simulink model "PID_Closed_Loop_2"  (R2023b)
settings: Solver=VariableStepAuto  StartTime=0.0  StopTime=100  FixedStep=0.1  RelTol=1e-05
values from neighbouring files (symbols this model uses):
  F_max = 1.0    (= 1)    [Parameters.m]    (also in Parameters_.m)
  J = 1    [Parameters.m]    (also in Parameters_.m = 0.0178)
  Kd = 5    [Parameters.m]    (also in Parameters_.m = 8)
  KI = 5    [Parameters.m]    (also in Parameters_.m = 2)
  Kp = 8    [Parameters.m]    (also in Parameters_.m)
  L = 0.160    (= 0.16)    [Parameters.m]    (also in Parameters_.m = 0.41)
  m = 2    [Parameters.m]    (also in Parameters_.m = 2.05)
  r = 0.033    [Parameters.m]    (also in Parameters_.m = 0.1)
libraries: slpidlib x2
settings Model: Creator=yosse  LastModifiedBy=DELL
settings DebuggingCC: AlgebraicLoopMsg=none

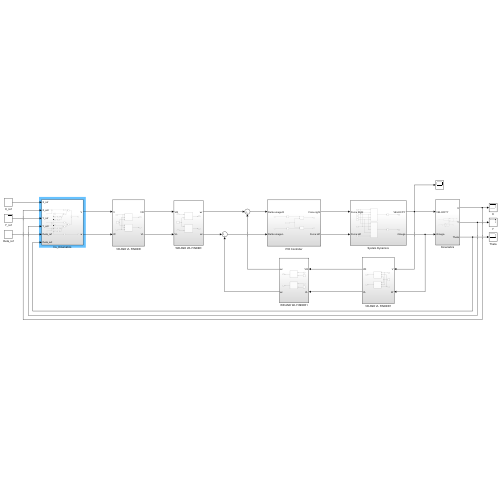
[thumbnail: Simulink's stored preview of the top-level diagram]
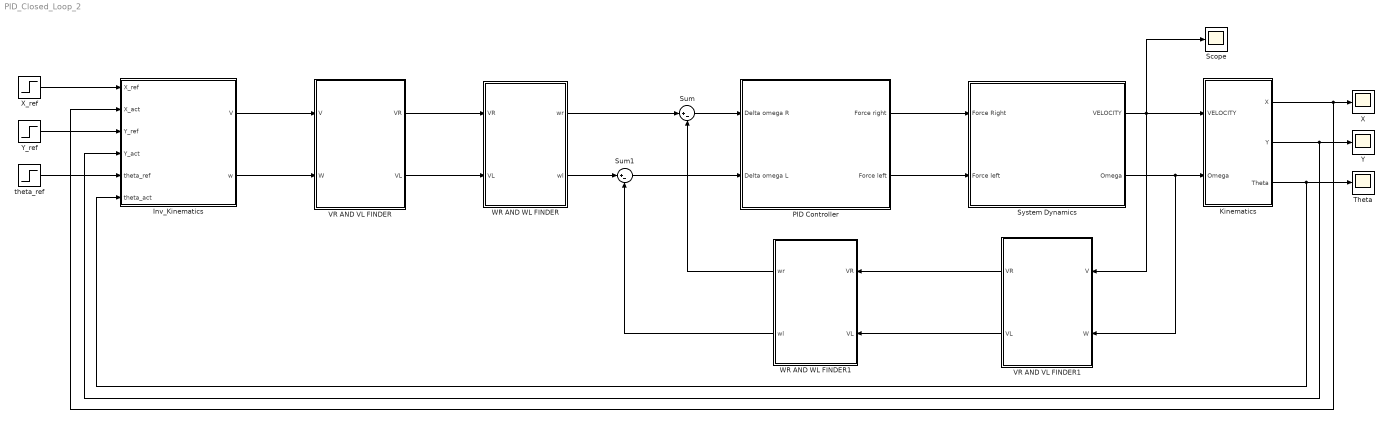
== system PID_Closed_Loop_2 ==
  Inv_Kinematics : Subsystem
  Kinematics : Subsystem
  PID Controller : Subsystem
  Scope : Scope
  Sum : Sum  Inputs=|+-
  Sum1 : Sum  Inputs=|+-
  System Dynamics : Subsystem
  Theta : Scope
  VR AND VL FINDER : Subsystem
  VR AND VL FINDER1 : Subsystem
  WR AND WL FINDER : Subsystem
  WR AND WL FINDER1 : Subsystem
  X : Scope
  X_ref : Step  SampleTime=0
  Y : Scope
  Y_ref : Step  After=0  SampleTime=0
  theta_ref : Step  After=0  SampleTime=0
  wires:
  System Dynamics/2(Omega) -> VR AND VL FINDER1/2(W), Kinematics/2(Omega)
  System Dynamics/1(VELOCITY) -> Scope/1, VR AND VL FINDER1/1(V), Kinematics/1(VELOCITY)
  PID Controller/2(Force left) -> System Dynamics/2(Force left)
  PID Controller/1(Force right) -> System Dynamics/1(Force Right)
  VR AND VL FINDER/1(VR) -> WR AND WL FINDER/1(VR)
  VR AND VL FINDER/2(VL) -> WR AND WL FINDER/2(VL)
  Kinematics/1(X) -> Inv_Kinematics/2(X_act), X/1
  Kinematics/2(Y) -> Inv_Kinematics/4(Y_act), Y/1
  Kinematics/3(Theta) -> Inv_Kinematics/6(theta_act), Theta/1
  VR AND VL FINDER1/1(VR) -> WR AND WL FINDER1/1(VR)
  VR AND VL FINDER1/2(VL) -> WR AND WL FINDER1/2(VL)
  WR AND WL FINDER/1(wr) -> Sum/1
  WR AND WL FINDER/2(wl) -> Sum1/1
  Sum1/1 -> PID Controller/2(Delta omega L)
  Sum/1 -> PID Controller/1(Delta omega R)
  WR AND WL FINDER1/1(wr) -> Sum/2
  WR AND WL FINDER1/2(wl) -> Sum1/2
  Inv_Kinematics/1(V) -> VR AND VL FINDER/1(V)
  Inv_Kinematics/2(w) -> VR AND VL FINDER/2(W)
  X_ref/1 -> Inv_Kinematics/1(X_ref)
  Y_ref/1 -> Inv_Kinematics/3(Y_ref)
  theta_ref/1 -> Inv_Kinematics/5(theta_ref)

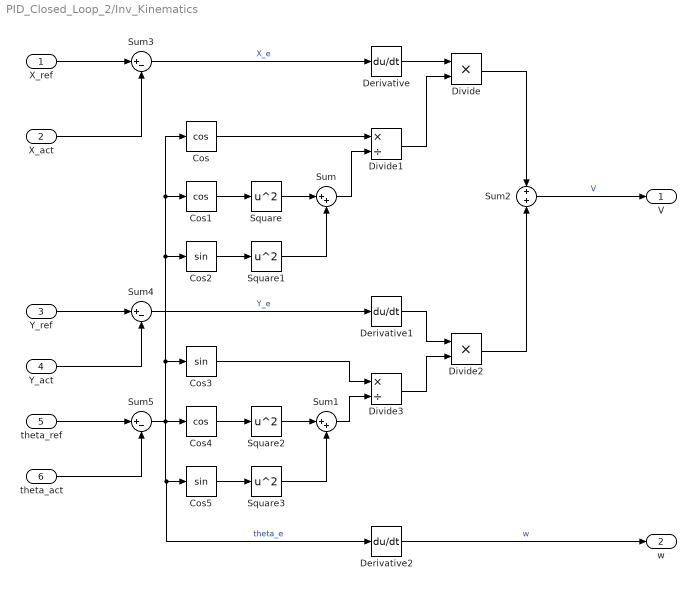
== system PID_Closed_Loop_2/Inv_Kinematics ==
  X_ref : Inport
  X_act : Inport  Port=2
  Y_ref : Inport  Port=3
  Y_act : Inport  Port=4
  theta_ref : Inport  Port=5
  theta_act : Inport  Port=6
  Cos : Trigonometry  Operator=cos
  Cos1 : Trigonometry  Operator=cos
  Cos2 : Trigonometry
  Cos3 : Trigonometry
  Cos4 : Trigonometry  Operator=cos
  Cos5 : Trigonometry
  Derivative : Derivative
  Derivative1 : Derivative
  Derivative2 : Derivative
  Divide : Product  Inputs=**
  Divide1 : Product  Inputs=*/
  Divide2 : Product  Inputs=**
  Divide3 : Product  Inputs=*/
  Square{,1..3} (4 alike) : Math  Operator=square
  Sum : Sum  Inputs=|++
  Sum1 : Sum  Inputs=|++
  Sum2 : Sum  Inputs=+|+
  Sum3 : Sum  Inputs=|+-
  Sum4 : Sum  Inputs=|+-
  Sum5 : Sum  Inputs=|+-
  V : Outport
  w : Outport  Port=2
  wires:
  Sum2/1 -> V/1  "V"
  Divide/1 -> Sum2/1
  Square2/1 -> Sum1/1
  Sum/1 -> Divide1/2
  Divide2/1 -> Sum2/2
  Cos1/1 -> Square/1
  Divide3/1 -> Divide2/2
  Derivative/1 -> Divide/1
  Cos/1 -> Divide1/1
  Square1/1 -> Sum/2
  Cos3/1 -> Divide3/1
  Divide1/1 -> Divide/2
  Square/1 -> Sum/1
  Cos5/1 -> Square3/1
  Sum1/1 -> Divide3/2
  Cos4/1 -> Square2/1
  Square3/1 -> Sum1/2
  Cos2/1 -> Square1/1
  Derivative1/1 -> Divide2/1
  Derivative2/1 -> w/1  "w"
  X_ref/1 -> Sum3/1
  Sum3/1 -> Derivative/1  "X_e"
  Y_ref/1 -> Sum4/1
  Sum4/1 -> Derivative1/1  "Y_e"
  Sum5/1 -> Cos2/1, Cos/1, Cos1/1, Cos3/1, Derivative2/1, Cos5/1, Cos4/1  "theta_e"
  theta_ref/1 -> Sum5/1
  X_act/1 -> Sum3/2
  Y_act/1 -> Sum4/2
  theta_act/1 -> Sum5/2

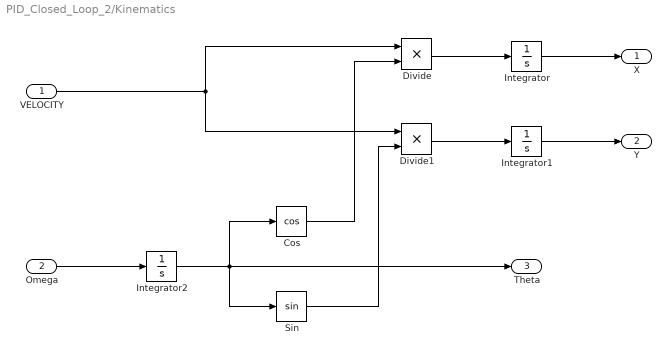
== system PID_Closed_Loop_2/Kinematics ==
  VELOCITY : Inport
  Omega : Inport  Port=2
  Cos : Trigonometry  Operator=cos
  Divide : Product  Inputs=**
  Divide1 : Product  Inputs=**
  Integrator : Integrator
  Integrator1 : Integrator
  Integrator2 : Integrator
  Sin : Trigonometry
  X : Outport
  Y : Outport  Port=2
  Theta : Outport  Port=3
  wires:
  Divide1/1 -> Integrator1/1
  Sin/1 -> Divide1/2
  Integrator2/1 -> Theta/1, Cos/1, Sin/1
  Cos/1 -> Divide/2
  Divide/1 -> Integrator/1
  Integrator/1 -> X/1
  Integrator1/1 -> Y/1
  Omega/1 -> Integrator2/1
  VELOCITY/1 -> Divide1/1, Divide/1

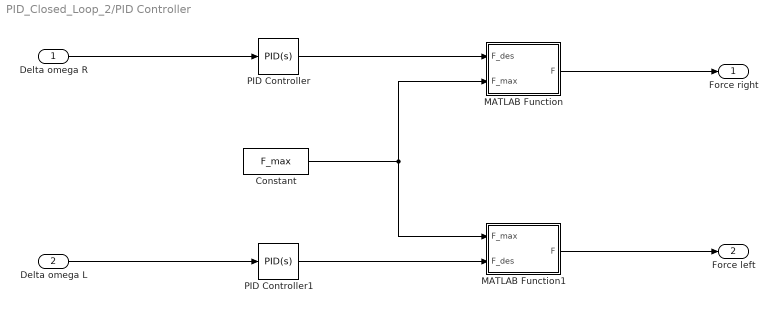
== system PID_Closed_Loop_2/PID Controller ==
  Delta omega R : Inport
  Delta omega L : Inport  Port=2
  Constant : Constant  Value=F_max
  MATLAB Function : MATLAB Function  TreatAsAtomicUnit=on
  MATLAB Function1 : MATLAB Function  TreatAsAtomicUnit=on
  PID Controller : slpidlib/PID Controller  Controller=PID  Form=Parallel  TimeDomain=Continuous-time  UseExternalTs=off  SampleTime=-1  IntegratorMethod=Forward Euler  FilterMethod=Forward Euler  ControllerParametersSource=internal  P=Kp  I=KI  UseKiTs=off  D=Kd  N=100  UseFilter=on  TunerSelectOption=Transfer Function Based (PID Tuner App)  InitialConditionSource=internal  InitialConditionForIntegrator=0  InitialConditionForFilter=0  DifferentiatorICPrevScaledInput=0  ExternalReset=none  TrackingMode=off  Kt=1  LimitOutput=off  SatLimitsSource=internal  UpperSaturationLimit=inf  LowerSaturationLimit=-inf  LinearizeAsGain=on  AntiWindupMode=none  Kb=1  LimitIntegrator=off  UpperIntegratorSaturationLimit=inf  LowerIntegratorSaturationLimit=-inf  POutMin=[]  POutMax=[]  IOutMin=[]  IOutMax=[]  DOutMin=[]  DOutMax=[]  NOutMin=[]  NOutMax=[]  SumOutMin=[]  SumOutMax=[]  SaturationOutMin=[]  SaturationOutMax=[]  PParamMin=[]  PParamMax=[]  IParamMin=[]  IParamMax=[]  DParamMin=[]  DParamMax=[]  NParamMin=[]  NParamMax=[]  KbParamMin=[]  KbParamMax=[]  KtParamMin=[]  KtParamMax=[]  KbOutMin=[]  KbOutMax=[]  KtOutMin=[]  KtOutMax=[]  IntegratorOutMin=[]  IntegratorOutMax=[]  FilterOutMin=[]  FilterOutMax=[]  SumI1OutMin=[]  SumI1OutMax=[]  SumI2OutMin=[]  SumI2OutMax=[]  SumI3OutMin=[]  SumI3OutMax=[]  SumI4OutMin=[]  SumI4OutMax=[]  SumDOutMin=[]  SumDOutMax=[]  DifferentiatorOutMin=[]  DifferentiatorOutMax=[]  FilterDiffOutCoefMin=[]  FilterDiffOutCoefMax=[]  ReciprocalOutMin=[]  ReciprocalOutMax=[]  SumDenOutMin=[]  SumDenOutMax=[]  SumNumOutMin=[]  SumNumOutMax=[]  DivideOutMin=[]  DivideOutMax=[]  UdiffTsProdOutMin=[]  UdiffTsProdOutMax=[]  NTsProdOutMin=[]  NTsProdOutMax=[]  UintegralTsProdOutMin=[]  UintegralTsProdOutMax=[]  UngainTsProdOutMin=[]  UngainTsProdOutMax=[]  ClampingZeroOutDataTypeStr=Inherit: Inherit via back propagation  ClampingZeroOutMin=[]  ClampingZeroOutMax=[]  FilterDenConstantOutDataTypeStr=Inherit: Inherit via back propagation  FilterDenConstantOutMin=[]  FilterDenConstantOutMax=[]  PCopyOutDataTypeStr=Inherit: Inherit via back propagation  PCopyOutMin=[]  PCopyOutMax=[]  NCopyOutDataTypeStr=Inherit: Inherit via back propagation  NCopyOutMin=[]  NCopyOutMax=[]  IntegratorContinuousStateAttributes=''  IntegratorStateMustResolveToSignalObject=off  IntegratorRTWStateStorageClass=Auto  FilterContinuousStateAttributes=''  FilterStateMustResolveToSignalObject=off  FilterRTWStateStorageClass=Auto  ParallelPVariant=InternalParameters  IdealPVariant=Disabled  IVariant=InternalParameters  DVariant=InternalParameters  IntegratorVariant=Continuous  SatVariant=Disabled  AWVariant=Passthrough  PCopyVariant=Disabled  TRVariant=Disabled  FdbkBlocksVariant=Forward  IdealPFdbkVariant=Disabled  SatFdbkVariant=Disabled  DerivativeFilterVariant=ContFilter  NVariant=InternalParameters  NCopyVariant=Disabled  FilterICVariant=InternalICsFilter  IntegratorICVariant=InternalICs  ExternalResetVariant=Disabled  TRSumVariant=Passthrough  SumFdbkVariant=Disabled  SumVariant=Sum_PID  TsampFilterVariant=InternalTs  TsampNgainVariant=Passthrough  TsampIntegralVariant=Disabled_SignalSpec  ExternalSaturationOutDataTypeStr=Inherit: Same as second input
  PID Controller1 : slpidlib/PID Controller  Controller=PID  Form=Parallel  TimeDomain=Continuous-time  UseExternalTs=off  SampleTime=-1  IntegratorMethod=Forward Euler  FilterMethod=Forward Euler  ControllerParametersSource=internal  P=Kp  I=KI  UseKiTs=off  D=Kd  N=100  UseFilter=on  TunerSelectOption=Transfer Function Based (PID Tuner App)  InitialConditionSource=internal  InitialConditionForIntegrator=0  InitialConditionForFilter=0  DifferentiatorICPrevScaledInput=0  ExternalReset=none  TrackingMode=off  Kt=1  LimitOutput=off  SatLimitsSource=internal  UpperSaturationLimit=inf  LowerSaturationLimit=-inf  LinearizeAsGain=on  AntiWindupMode=none  Kb=1  LimitIntegrator=off  UpperIntegratorSaturationLimit=inf  LowerIntegratorSaturationLimit=-inf  POutMin=[]  POutMax=[]  IOutMin=[]  IOutMax=[]  DOutMin=[]  DOutMax=[]  NOutMin=[]  NOutMax=[]  SumOutMin=[]  SumOutMax=[]  SaturationOutMin=[]  SaturationOutMax=[]  PParamMin=[]  PParamMax=[]  IParamMin=[]  IParamMax=[]  DParamMin=[]  DParamMax=[]  NParamMin=[]  NParamMax=[]  KbParamMin=[]  KbParamMax=[]  KtParamMin=[]  KtParamMax=[]  KbOutMin=[]  KbOutMax=[]  KtOutMin=[]  KtOutMax=[]  IntegratorOutMin=[]  IntegratorOutMax=[]  FilterOutMin=[]  FilterOutMax=[]  SumI1OutMin=[]  SumI1OutMax=[]  SumI2OutMin=[]  SumI2OutMax=[]  SumI3OutMin=[]  SumI3OutMax=[]  SumI4OutMin=[]  SumI4OutMax=[]  SumDOutMin=[]  SumDOutMax=[]  DifferentiatorOutMin=[]  DifferentiatorOutMax=[]  FilterDiffOutCoefMin=[]  FilterDiffOutCoefMax=[]  ReciprocalOutMin=[]  ReciprocalOutMax=[]  SumDenOutMin=[]  SumDenOutMax=[]  SumNumOutMin=[]  SumNumOutMax=[]  DivideOutMin=[]  DivideOutMax=[]  UdiffTsProdOutMin=[]  UdiffTsProdOutMax=[]  NTsProdOutMin=[]  NTsProdOutMax=[]  UintegralTsProdOutMin=[]  UintegralTsProdOutMax=[]  UngainTsProdOutMin=[]  UngainTsProdOutMax=[]  ClampingZeroOutDataTypeStr=Inherit: Inherit via back propagation  ClampingZeroOutMin=[]  ClampingZeroOutMax=[]  FilterDenConstantOutDataTypeStr=Inherit: Inherit via back propagation  FilterDenConstantOutMin=[]  FilterDenConstantOutMax=[]  PCopyOutDataTypeStr=Inherit: Inherit via back propagation  PCopyOutMin=[]  PCopyOutMax=[]  NCopyOutDataTypeStr=Inherit: Inherit via back propagation  NCopyOutMin=[]  NCopyOutMax=[]  IntegratorContinuousStateAttributes=''  IntegratorStateMustResolveToSignalObject=off  IntegratorRTWStateStorageClass=Auto  FilterContinuousStateAttributes=''  FilterStateMustResolveToSignalObject=off  FilterRTWStateStorageClass=Auto  ParallelPVariant=InternalParameters  IdealPVariant=Disabled  IVariant=InternalParameters  DVariant=InternalParameters  IntegratorVariant=Continuous  SatVariant=Disabled  AWVariant=Passthrough  PCopyVariant=Disabled  TRVariant=Disabled  FdbkBlocksVariant=Forward  IdealPFdbkVariant=Disabled  SatFdbkVariant=Disabled  DerivativeFilterVariant=ContFilter  NVariant=InternalParameters  NCopyVariant=Disabled  FilterICVariant=InternalICsFilter  IntegratorICVariant=InternalICs  ExternalResetVariant=Disabled  TRSumVariant=Passthrough  SumFdbkVariant=Disabled  SumVariant=Sum_PID  TsampFilterVariant=InternalTs  TsampNgainVariant=Passthrough  TsampIntegralVariant=Disabled_SignalSpec  ExternalSaturationOutDataTypeStr=Inherit: Same as second input
  Force right : Outport
  Force left : Outport  Port=2
  wires:
  Delta omega R/1 -> PID Controller/1
  Delta omega L/1 -> PID Controller1/1
  PID Controller/1 -> MATLAB Function/1(F_des)
  MATLAB Function/1(F) -> Force right/1
  PID Controller1/1 -> MATLAB Function1/2(F_des)
  MATLAB Function1/1(F) -> Force left/1
  Constant/1 -> MATLAB Function1/1(F_max), MATLAB Function/2(F_max)

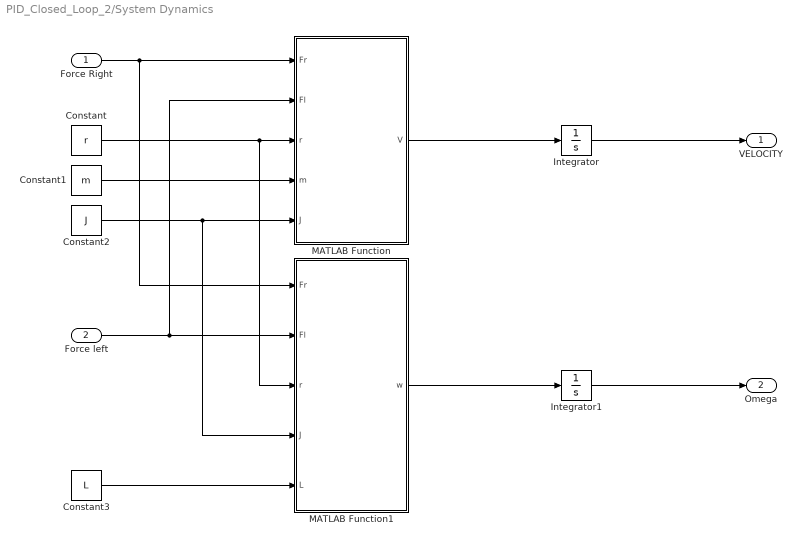
== system PID_Closed_Loop_2/System Dynamics ==
  Force Right : Inport
  Force left : Inport  Port=2
  Constant : Constant  Value=r
  Constant1 : Constant  Value=m
  Constant2 : Constant  Value=J
  Constant3 : Constant  Value=L
  Integrator : Integrator
  Integrator1 : Integrator
  MATLAB Function : MATLAB Function  TreatAsAtomicUnit=on
  MATLAB Function1 : MATLAB Function  TreatAsAtomicUnit=on
  VELOCITY : Outport
  Omega : Outport  Port=2
  wires:
  MATLAB Function/1(V) -> Integrator/1
  Force Right/1 -> MATLAB Function1/1(Fr), MATLAB Function/1(Fr)
  Force left/1 -> MATLAB Function/2(Fl), MATLAB Function1/2(Fl)
  MATLAB Function1/1(w) -> Integrator1/1
  Constant/1 -> MATLAB Function1/3(r), MATLAB Function/3(r)
  Constant1/1 -> MATLAB Function/4(m)
  Constant2/1 -> MATLAB Function1/4(J), MATLAB Function/5(J)
  Constant3/1 -> MATLAB Function1/5(L)
  Integrator/1 -> VELOCITY/1
  Integrator1/1 -> Omega/1

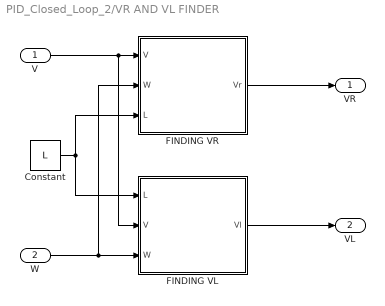
== system PID_Closed_Loop_2/VR AND VL FINDER ==
  V : Inport
  W : Inport  Port=2
  Constant : Constant  Value=L
  FINDING VL : MATLAB Function  TreatAsAtomicUnit=on
  FINDING VR : MATLAB Function  TreatAsAtomicUnit=on
  VR : Outport
  VL : Outport  Port=2
  wires:
  V/1 -> FINDING VL/2(V), FINDING VR/1(V)
  W/1 -> FINDING VR/2(W), FINDING VL/3(W)
  FINDING VR/1(Vr) -> VR/1
  FINDING VL/1(Vl) -> VL/1
  Constant/1 -> FINDING VR/3(L), FINDING VL/1(L)

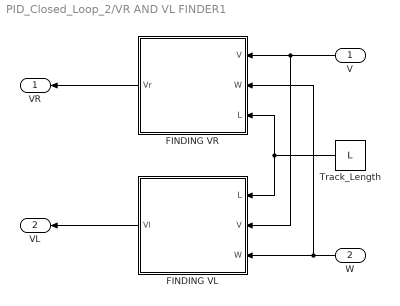
== system PID_Closed_Loop_2/VR AND VL FINDER1 ==
  V : Inport
  W : Inport  Port=2
  FINDING VL : MATLAB Function  TreatAsAtomicUnit=on
  FINDING VR : MATLAB Function  TreatAsAtomicUnit=on
  Track_Length : Constant  Value=L
  VR : Outport
  VL : Outport  Port=2
  wires:
  V/1 -> FINDING VL/2(V), FINDING VR/1(V)
  W/1 -> FINDING VR/2(W), FINDING VL/3(W)
  FINDING VR/1(Vr) -> VR/1
  FINDING VL/1(Vl) -> VL/1
  Track_Length/1 -> FINDING VR/3(L), FINDING VL/1(L)

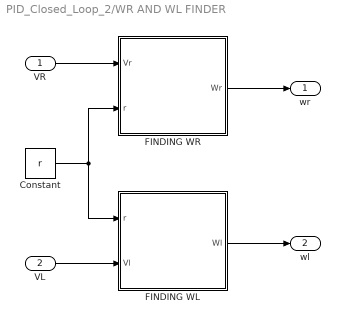
== system PID_Closed_Loop_2/WR AND WL FINDER ==
  VR : Inport
  VL : Inport  Port=2
  Constant : Constant  Value=r
  FINDING WL : MATLAB Function  TreatAsAtomicUnit=on
  FINDING WR : MATLAB Function  TreatAsAtomicUnit=on
  wr : Outport
  wl : Outport  Port=2
  wires:
  FINDING WR/1(Wr) -> wr/1
  FINDING WL/1(Wl) -> wl/1
  VR/1 -> FINDING WR/1(Vr)
  VL/1 -> FINDING WL/2(Vl)
  Constant/1 -> FINDING WL/1(r), FINDING WR/2(r)

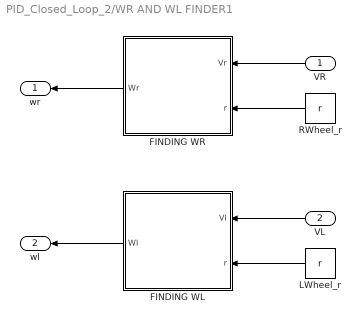
== system PID_Closed_Loop_2/WR AND WL FINDER1 ==
  VR : Inport
  VL : Inport  Port=2
  FINDING WL : MATLAB Function  TreatAsAtomicUnit=on
  FINDING WR : MATLAB Function  TreatAsAtomicUnit=on
  LWheel_r : Constant  Value=r
  RWheel_r : Constant  Value=r
  wr : Outport
  wl : Outport  Port=2
  wires:
  FINDING WR/1(Wr) -> wr/1
  FINDING WL/1(Wl) -> wl/1
  VR/1 -> FINDING WR/1(Vr)
  VL/1 -> FINDING WL/1(Vl)
  RWheel_r/1 -> FINDING WR/2(r)
  LWheel_r/1 -> FINDING WL/2(r)

== matlab function PID_Closed_Loop_2/VR AND VL FINDER1/FINDING VR ==
  data: V input; Vr output; W input; L input
function Vr = fcn(V,W, L)

Vr = V + ((L/2)*W);

== matlab function PID_Closed_Loop_2/System Dynamics/MATLAB Function1 ==
  data: Fr input; Fl input; r input; J input; L input; w output
function w = fcn(Fr, Fl, r, J, L)

%v = (Fr-Fl) * L;
%x = (2 * J) + (J * (L^2)/(r^2));

w = ((Fr - Fl) * L) / ((2 * J) + (J * (L^2)/(r^2)));

== matlab function PID_Closed_Loop_2/System Dynamics/MATLAB Function ==
  data: Fr input; V output; Fl input; r input; m input; J input
function V = fcn(Fr, Fl, r, m, J)

%v = (Fr+Fl);
%x = (2*J/(33^2)) + (m);

V = (Fr + Fl) / ((2*J/(r^2)) + (m));

== matlab function PID_Closed_Loop_2/VR AND VL FINDER/FINDING VR ==
  data: V input; Vr output; W input; L input
function Vr = fcn(V, W, L)

Vr = V + ((L/2) * W);

== matlab function PID_Closed_Loop_2/VR AND VL FINDER/FINDING VL ==
  data: L input; V input; Vl output; W input
function Vl = fcn(L, V, W)

Vl = V - ((L/2) * W);

== matlab function PID_Closed_Loop_2/WR AND WL FINDER/FINDING WL ==
  data: r input; Vl input; Wl output
function Wl = fcn(r, Vl)

Wl = (Vl/r);

== matlab function PID_Closed_Loop_2/WR AND WL FINDER/FINDING WR ==
  data: Vr input; Wr output; r input
function Wr = fcn(Vr, r)

Wr = (Vr/r);

== matlab function PID_Closed_Loop_2/PID Controller/MATLAB Function ==
  data: F_des input; F output; F_max input
function F = fcn(F_des, F_max)

if abs(F_des) > F_max
    if F_des >= 0
        F = F_max;
    else
        F = -F_max;
    end

else
    F = F_des;
end

== matlab function PID_Closed_Loop_2/PID Controller/MATLAB Function1 ==
  data: F_max input; F_des input; F output
function F = fcn(F_max, F_des)

if abs(F_des) > F_max
    if F_des >= 0
        F = F_max;
    else
        F = -F_max;
    end

else
    F = F_des;
end

== matlab function PID_Closed_Loop_2/WR AND WL FINDER1/FINDING WL ==
  data: Vl input; Wl output; r input
function Wl = fcn(Vl, r)

Wl = (Vl/r);

== matlab function PID_Closed_Loop_2/WR AND WL FINDER1/FINDING WR ==
  data: Vr input; Wr output; r input
function Wr = fcn(Vr, r)

Wr = (Vr/r);

== matlab function PID_Closed_Loop_2/VR AND VL FINDER1/FINDING VL ==
  data: L input; V input; Vl output; W input
function Vl = fcn(L,V,W)

Vl = V - ((L/2)*W);
